simulink model "Datapath"  (R2015a)
settings: Solver=ode45  StartTime=0.0  StopTime=10.0  RelTol=1e-3
settings Model: Creator=N1amr  LastModifiedBy=N1amr

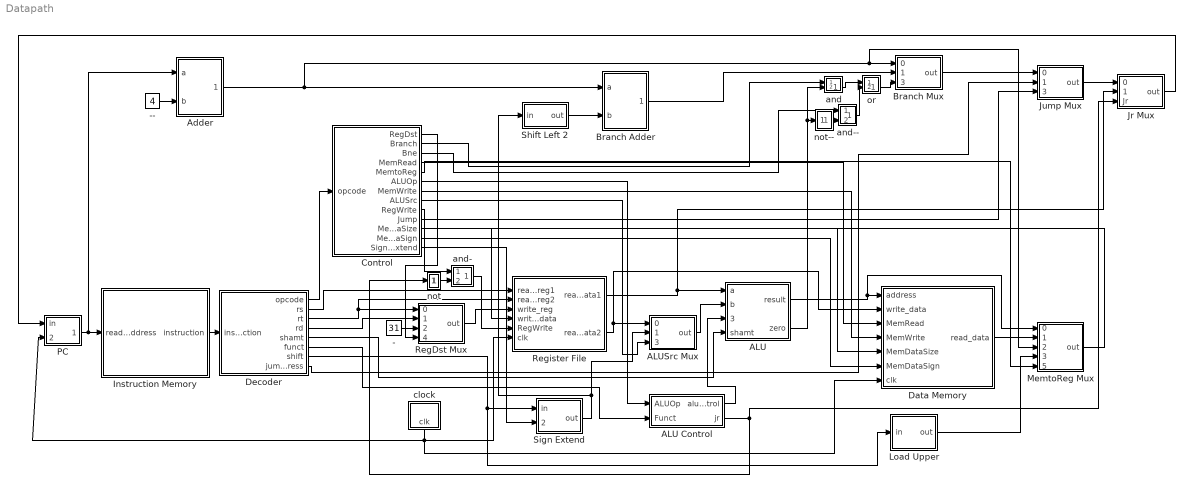
== system Datapath ==
  ALU : Subsystem
  ALU Control : Subsystem
  ALUSrc Mux : Subsystem
  Adder : Subsystem
  Branch Adder : Subsystem
  Branch Mux : Subsystem
  Control : Subsystem
  Data Memory : Subsystem
  Decoder : Subsystem
  Instruction Memory : Subsystem
  Jr Mux : Subsystem
  Jump Mux : Subsystem
  Load Upper : Subsystem
  MemtoReg Mux : Subsystem
  PC : Subsystem
  RegDst Mux : Subsystem
  Register File : Subsystem
  "Shift Left 2 " : Subsystem
  Sign Extend : Subsystem
  and : Subsystem
  and­ : Subsystem
  and­­ : Subsystem
  clock : Subsystem
  not : Subsystem
  not­­ : Subsystem
  or : Subsystem
  ­ : Constant  Value=31
  ­­ : Constant  Value=4
  wires:
  Instruction Memory/1(instruction) -> Decoder/1(instruction)
  Decoder/8(jump_address) -> Jump Mux/2(1)
  RegDst Mux/1(out) -> Register File/3(write_reg)
  Decoder/2(rs) -> Register File/1(read_reg1)
  Decoder/3(rt) -> Register File/2(read_reg2), RegDst Mux/1(0)
  Decoder/4(rd) -> RegDst Mux/2(1)
  Control/1(RegDst) -> RegDst Mux/4(RegDst)
  Register File/1(read_data1) -> Jr Mux/2(1), ALU/1(a)
  Control/8(ALUSrc) -> ALUSrc Mux/3(ALUSrc)
  Sign Extend/1(out) -> "Shift Left 2 "/1(in), ALUSrc Mux/2(1)
  Decoder/7(shift) -> Sign Extend/1(in), Load Upper/1(in)
  Decoder/5(shamt) -> ALU/4(shamt)
  Decoder/6(funct) -> ALU Control/2(Funct)
  Control/6(ALUOp) -> ALU Control/1(ALUOp)
  Control/4(MemRead) -> Data Memory/3(MemRead)
  Control/7(MemWrite) -> Data Memory/4(MemWrite)
  Data Memory/1(read_data) -> MemtoReg Mux/2(1)
  Control/5(MemtoReg) -> MemtoReg Mux/5(MemtoReg1)
  MemtoReg Mux/1(out) -> Register File/4(write_data)
  ­­/1 -> Adder/2(b)
  PC/1(out) -> Adder/1(a), Instruction Memory/1(read_address)
  "Shift Left 2 "/1(out) -> Branch Adder/2(b)
  Adder/1(result) -> Branch Mux/1(0), MemtoReg Mux/3(2), Branch Adder/1(a)
  Branch Adder/1(result) -> Branch Mux/2(1)
  Branch Mux/1(out) -> Jump Mux/1(0)
  Control/2(Branch) -> and/1(a)
  Decoder/1(opcode) -> Control/1(opcode)
  Register File/2(read_data2) -> Data Memory/2(write_data), ALUSrc Mux/1(0)
  ALUSrc Mux/1(out) -> ALU/2(b)
  ALU Control/1(alucontrol) -> ALU/3(alu_control)
  clock/1(clk) -> PC/2(clk), Data Memory/7(clk), Register File/6(clk)
  ALU/1(result) -> MemtoReg Mux/1(0), Data Memory/1(address)
  ­/1 -> RegDst Mux/3(2)
  not/1(out) -> and­/2(b)
  and­/1(f) -> Register File/5(RegWrite)
  ALU Control/2(jr) -> Jr Mux/3(Jr), not/1(in)
  Jump Mux/1(out) -> Jr Mux/1(0)
  Jr Mux/1(out) -> PC/1(in)
  Control/10(Jump) -> Jump Mux/3(Jump)
  Control/11(MemDataSize) -> Data Memory/5(MemDataSize)
  Control/12(MemDataSign) -> Data Memory/6(MemDataSign)
  Control/9(RegWrite) -> and­/1(a)
  Control/13(SignExtend) -> Sign Extend/2(sign)
  Control/3(Bne) -> and­­/1(a)
  and/1(f) -> or/1(a)
  or/1(f) -> Branch Mux/3(Take)
  and­­/1(f) -> or/2(b)
  not­­/1(f) -> and­­/2(b)
  ALU/2(zero) -> not­­/1(a), and/2(b)
  Load Upper/1(out) -> MemtoReg Mux/4(3)

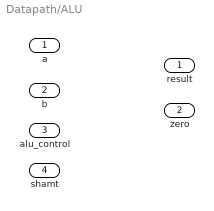
== system Datapath/ALU ==
  a : Inport
  b : Inport  Port=2
  alu_control : Inport  Port=3
  shamt : Inport  Port=4
  result : Outport
  zero : Outport  Port=2

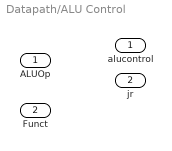
== system Datapath/ALU Control ==
  ALUOp : Inport  OutDataTypeStr=boolean  PortDimensions=32
  Funct : Inport  Port=2  PortDimensions=32
  alucontrol : Outport  PortDimensions=32
  jr : Outport  Port=2  PortDimensions=32

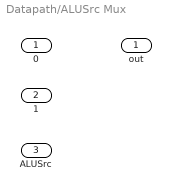
== system Datapath/ALUSrc Mux ==
  0 : Inport  OutDataTypeStr=boolean  PortDimensions=32
  1 : Inport  Port=2  PortDimensions=32
  ALUSrc : Inport  Port=3
  out : Outport  PortDimensions=32

== system Datapath/Adder ==
  a : Inport
  b : Inport  Port=2
  result : Outport

== system Datapath/Branch Adder ==
  a : Inport
  b : Inport  Port=2
  result : Outport

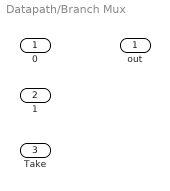
== system Datapath/Branch Mux ==
  0 : Inport  OutDataTypeStr=boolean  PortDimensions=32
  1 : Inport  Port=2  PortDimensions=32
  Take : Inport  Port=3
  out : Outport  PortDimensions=32

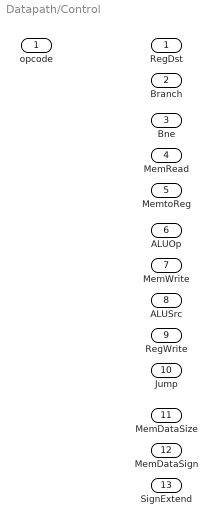
== system Datapath/Control ==
  opcode : Inport
  RegDst : Outport
  Branch : Outport  Port=2
  Bne : Outport  Port=3
  MemRead : Outport  Port=4
  MemtoReg : Outport  Port=5
  ALUOp : Outport  Port=6
  MemWrite : Outport  Port=7
  ALUSrc : Outport  Port=8
  RegWrite : Outport  Port=9
  Jump : Outport  Port=10
  MemDataSize : Outport  Port=11
  MemDataSign : Outport  Port=12
  SignExtend : Outport  Port=13

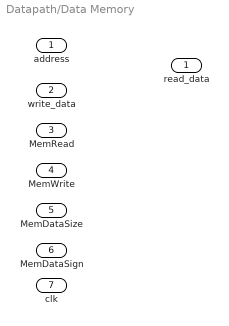
== system Datapath/Data Memory ==
  address : Inport
  write_data : Inport  Port=2
  MemRead : Inport  Port=3
  MemWrite : Inport  Port=4
  MemDataSize : Inport  Port=5
  MemDataSign : Inport  Port=6
  clk : Inport  Port=7
  read_data : Outport

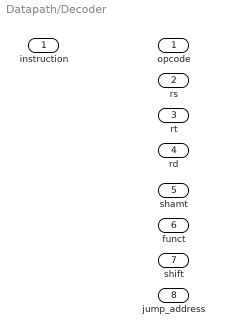
== system Datapath/Decoder ==
  instruction : Inport
  opcode : Outport
  rs : Outport  Port=2
  rt : Outport  Port=3
  rd : Outport  Port=4
  shamt : Outport  Port=5
  funct : Outport  Port=6
  shift : Outport  Port=7
  jump_address : Outport  Port=8

== system Datapath/Instruction Memory ==
  read_address : Inport
  instruction : Outport

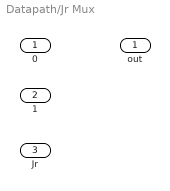
== system Datapath/Jr Mux ==
  0 : Inport  OutDataTypeStr=boolean  PortDimensions=32
  1 : Inport  Port=2  PortDimensions=32
  Jr : Inport  Port=3
  out : Outport  PortDimensions=32

== system Datapath/Jump Mux ==
  0 : Inport  OutDataTypeStr=boolean  PortDimensions=32
  1 : Inport  Port=2  PortDimensions=32
  Jump : Inport  Port=3
  out : Outport  PortDimensions=32

== system Datapath/Load Upper ==
  in : Inport  OutDataTypeStr=boolean  PortDimensions=32
  out : Outport  PortDimensions=32

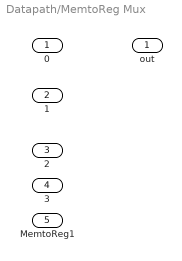
== system Datapath/MemtoReg Mux ==
  0 : Inport  OutDataTypeStr=boolean  PortDimensions=32
  1 : Inport  Port=2  PortDimensions=32
  2 : Inport  Port=3
  3 : Inport  Port=4
  MemtoReg1 : Inport  Port=5
  out : Outport  PortDimensions=32

== system Datapath/PC ==
  in : Inport
  clk : Inport  Port=2
  out : Outport

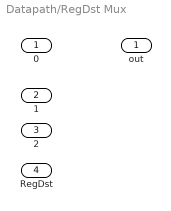
== system Datapath/RegDst Mux ==
  0 : Inport  OutDataTypeStr=boolean  PortDimensions=32
  1 : Inport  Port=2  PortDimensions=32
  2 : Inport  Port=3  PortDimensions=32
  RegDst : Inport  Port=4
  out : Outport  PortDimensions=32

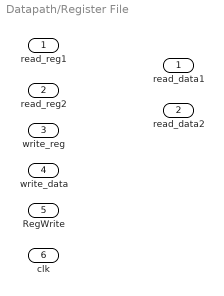
== system Datapath/Register File ==
  read_reg1 : Inport
  read_reg2 : Inport  Port=2
  write_reg : Inport  Port=3
  write_data : Inport  Port=4
  RegWrite : Inport  Port=5
  clk : Inport  Port=6
  read_data1 : Outport
  read_data2 : Outport  Port=2

== system Datapath/Shift Left 2  ==
  in : Inport  OutDataTypeStr=boolean  PortDimensions=32
  out : Outport  PortDimensions=32

== system Datapath/Sign Extend ==
  in : Inport  OutDataTypeStr=boolean  PortDimensions=32
  sign : Inport  Port=2
  out : Outport  PortDimensions=32

== system Datapath/and ==
  a : Inport  OutDataTypeStr=boolean  PortDimensions=32
  b : Inport  Port=2  PortDimensions=32
  f : Outport  PortDimensions=32

== system Datapath/and­ ==
  a : Inport  OutDataTypeStr=boolean  PortDimensions=32
  b : Inport  Port=2  PortDimensions=32
  f : Outport  PortDimensions=32

== system Datapath/and­­ ==
  a : Inport  OutDataTypeStr=boolean  PortDimensions=32
  b : Inport  Port=2  PortDimensions=32
  f : Outport  PortDimensions=32

== system Datapath/clock ==
  clk : Outport

== system Datapath/not ==
  in : Inport  OutDataTypeStr=boolean  PortDimensions=32
  out : Outport  PortDimensions=32

== system Datapath/not­­ ==
  a : Inport  OutDataTypeStr=boolean  PortDimensions=32
  f : Outport  PortDimensions=32

== system Datapath/or ==
  a : Inport  OutDataTypeStr=boolean  PortDimensions=32
  b : Inport  Port=2  PortDimensions=32
  f : Outport  PortDimensions=32
